simulink model "input_output_Linearization"  (R2015a)
settings: Solver=ode45  StartTime=0.0  StopTime=10.0  RelTol=1e-3
settings Model: Creator=root  LastModifiedBy=root

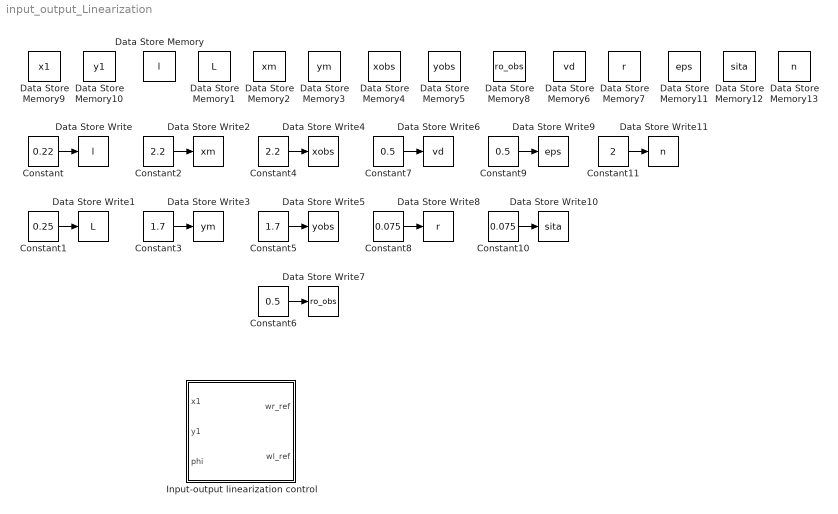
== system input_output_Linearization ==
  Constant : Constant  Value=0.22
  Constant1 : Constant  Value=0.25
  Constant10 : Constant  Value=0.075
  Constant11 : Constant  Value=2
  Constant2 : Constant  Value=2.2
  Constant3 : Constant  Value=1.7
  Constant4 : Constant  Value=2.2
  Constant5 : Constant  Value=1.7
  Constant6 : Constant  Value=0.5
  Constant7 : Constant  Value=0.5
  Constant8 : Constant  Value=0.075
  Constant9 : Constant  Value=0.5
  Data Store Memory : DataStoreMemory  DataStoreName=l  ReadBeforeWriteMsg=warning  WriteAfterWriteMsg=warning  WriteAfterReadMsg=warning
  Data Store Memory1 : DataStoreMemory  DataStoreName=L  ReadBeforeWriteMsg=warning  WriteAfterWriteMsg=warning  WriteAfterReadMsg=warning
  Data Store Memory10 : DataStoreMemory  DataStoreName=y1  ReadBeforeWriteMsg=warning  WriteAfterWriteMsg=warning  WriteAfterReadMsg=warning
  Data Store Memory11 : DataStoreMemory  DataStoreName=eps  ReadBeforeWriteMsg=warning  WriteAfterWriteMsg=warning  WriteAfterReadMsg=warning
  Data Store Memory12 : DataStoreMemory  DataStoreName=sita  ReadBeforeWriteMsg=warning  WriteAfterWriteMsg=warning  WriteAfterReadMsg=warning
  Data Store Memory13 : DataStoreMemory  DataStoreName=n  ReadBeforeWriteMsg=warning  WriteAfterWriteMsg=warning  WriteAfterReadMsg=warning
  Data Store Memory2 : DataStoreMemory  DataStoreName=xm  ReadBeforeWriteMsg=warning  WriteAfterWriteMsg=warning  WriteAfterReadMsg=warning
  Data Store Memory3 : DataStoreMemory  DataStoreName=ym  ReadBeforeWriteMsg=warning  WriteAfterWriteMsg=warning  WriteAfterReadMsg=warning
  Data Store Memory4 : DataStoreMemory  DataStoreName=xobs  ReadBeforeWriteMsg=warning  WriteAfterWriteMsg=warning  WriteAfterReadMsg=warning
  Data Store Memory5 : DataStoreMemory  DataStoreName=yobs  ReadBeforeWriteMsg=warning  WriteAfterWriteMsg=warning  WriteAfterReadMsg=warning
  Data Store Memory6 : DataStoreMemory  DataStoreName=vd  ReadBeforeWriteMsg=warning  WriteAfterWriteMsg=warning  WriteAfterReadMsg=warning
  Data Store Memory7 : DataStoreMemory  DataStoreName=r  ReadBeforeWriteMsg=warning  WriteAfterWriteMsg=warning  WriteAfterReadMsg=warning
  Data Store Memory8 : DataStoreMemory  DataStoreName=ro_obs  ReadBeforeWriteMsg=warning  WriteAfterWriteMsg=warning  WriteAfterReadMsg=warning
  Data Store Memory9 : DataStoreMemory  DataStoreName=x1  ReadBeforeWriteMsg=warning  WriteAfterWriteMsg=warning  WriteAfterReadMsg=warning
  Data Store Write : DataStoreWrite  DataStoreName=l
  Data Store Write1 : DataStoreWrite  DataStoreName=L
  Data Store Write10 : DataStoreWrite  DataStoreName=sita
  Data Store Write11 : DataStoreWrite  DataStoreName=n
  Data Store Write2 : DataStoreWrite  DataStoreName=xm
  Data Store Write3 : DataStoreWrite  DataStoreName=ym
  Data Store Write4 : DataStoreWrite  DataStoreName=xobs
  Data Store Write5 : DataStoreWrite  DataStoreName=yobs
  Data Store Write6 : DataStoreWrite  DataStoreName=vd
  Data Store Write7 : DataStoreWrite  DataStoreName=ro_obs
  Data Store Write8 : DataStoreWrite  DataStoreName=r
  Data Store Write9 : DataStoreWrite  DataStoreName=eps
  Input-output linearization control : Subsystem
  wires:
  Constant/1 -> Data Store Write/1
  Constant1/1 -> Data Store Write1/1
  Constant2/1 -> Data Store Write2/1
  Constant3/1 -> Data Store Write3/1
  Constant4/1 -> Data Store Write4/1
  Constant5/1 -> Data Store Write5/1
  Constant6/1 -> Data Store Write7/1
  Constant7/1 -> Data Store Write6/1
  Constant8/1 -> Data Store Write8/1
  Constant9/1 -> Data Store Write9/1
  Constant10/1 -> Data Store Write10/1
  Constant11/1 -> Data Store Write11/1

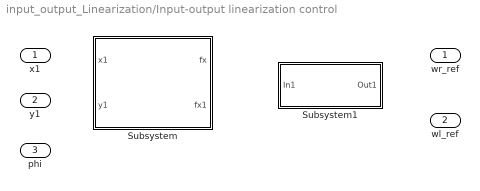
== system input_output_Linearization/Input-output linearization control ==
  x1 : Inport
  y1 : Inport  Port=2
  phi : Inport  Port=3
  Subsystem : Subsystem
  Subsystem1 : Subsystem
  wr_ref : Outport
  wl_ref : Outport  Port=2

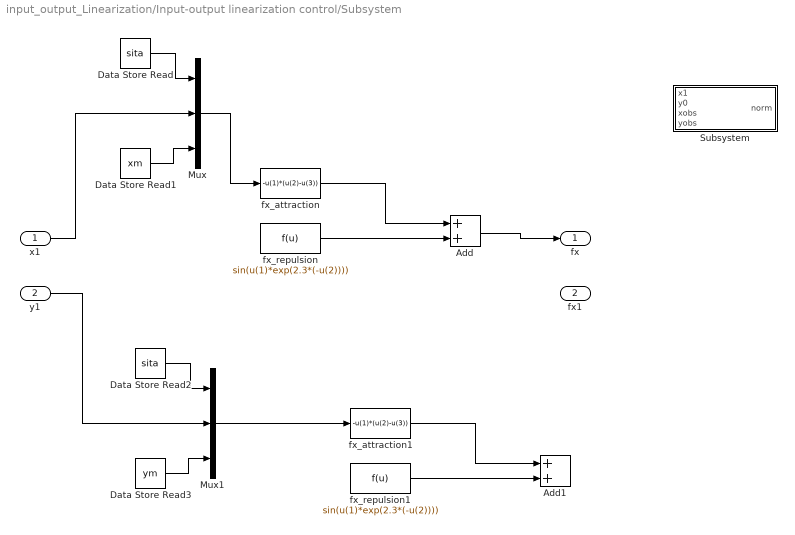
== system input_output_Linearization/Input-output linearization control/Subsystem ==
  x1 : Inport
  y1 : Inport  Port=2
  Add : Sum
  Add1 : Sum
  Data Store Read : DataStoreRead  DataStoreName=sita
  Data Store Read1 : DataStoreRead  DataStoreName=xm
  Data Store Read2 : DataStoreRead  DataStoreName=sita
  Data Store Read3 : DataStoreRead  DataStoreName=ym
  Mux : Mux  Inputs=3
  Mux1 : Mux  Inputs=3
  Subsystem : Subsystem
  fx_attraction : Fcn  Expr=-u(1)*(u(2)-u(3))
  fx_attraction1 : Fcn  Expr=-u(1)*(u(2)-u(3))
  fx_repulsion : Fcn  Expr=sin(u(1)*exp(2.3*(-u(2))))
  fx_repulsion1 : Fcn  Expr=sin(u(1)*exp(2.3*(-u(2))))
  fx : Outport
  fx1 : Outport  Port=2
  wires:
  fx_attraction/1 -> Add/1
  fx_repulsion/1 -> Add/2
  fx_attraction1/1 -> Add1/1
  fx_repulsion1/1 -> Add1/2
  Data Store Read/1 -> Mux/1
  Data Store Read1/1 -> Mux/3
  Mux/1 -> fx_attraction/1
  x1/1 -> Mux/2
  Data Store Read2/1 -> Mux1/1
  Data Store Read3/1 -> Mux1/3
  y1/1 -> Mux1/2
  Mux1/1 -> fx_attraction1/1
  Add/1 -> fx/1

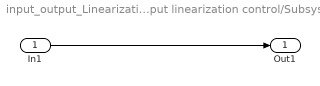
== system input_output_Linearization/Input-output linearization control/Subsystem1 ==
  In1 : Inport
  Out1 : Outport
  wires:
  In1/1 -> Out1/1

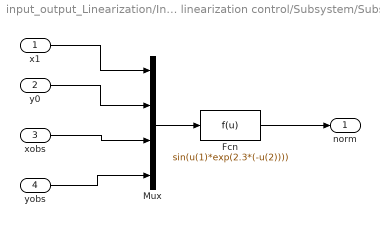
== system input_output_Linearization/Input-output linearization control/Subsystem/Subsystem ==
  x1 : Inport
  y0 : Inport  Port=2
  xobs : Inport  Port=3
  yobs : Inport  Port=4
  Fcn : Fcn  Expr=sin(u(1)*exp(2.3*(-u(2))))
  Mux : Mux
  norm : Outport
  wires:
  x1/1 -> Mux/1
  y0/1 -> Mux/2
  xobs/1 -> Mux/3
  yobs/1 -> Mux/4
  Mux/1 -> Fcn/1
  Fcn/1 -> norm/1
